simulink model "RefModel_Control"  (R2020b)
settings: Solver=ode1  StartTime=0.0  StopTime=1  FixedStep=0.012  MaxStep=Ts  RelTol=1e-3
settings Model: Creator=sl  LastModifiedBy=a4327481
settings DataIOCC: SaveOutput=off  SaveTime=off
settings OptimizationCC: DefaultParameterBehavior=Inlined  EnhancedBackFolding=on  PassReuseOutputArgsAs=Individual arguments  ZeroExternalMemoryAtStartup=off  ZeroInternalMemoryAtStartup=off  OptimizeBlockOrder=speed  DifferentSizesBufferReuse=on  OptimizationCustomize=off  EfficientTunableParamExpr=on
settings DebuggingCC: InheritedTsInSrcMsg=none  ParameterPrecisionLossMsg=none  ParameterTunabilityLossMsg=error  UnconnectedInputMsg=none  UnconnectedOutputMsg=none  UnconnectedLineMsg=none
settings HardwareCC: ProdBitPerPointer=32  ProdBitPerSizeT=32  ProdBitPerPtrDiffT=32  ProdLargestAtomicInteger=Long  ProdLargestAtomicFloat=Double  ProdWordSize=32  ProdHWDeviceType=ARM Compatible->ARM Cortex
settings ModelReferenceCC: ParallelModelReferenceMATLABWorkerInit=Copy Base Workspace  ModelReferenceNumInstancesAllowed=Single
settings SFSimCC: MATLABDynamicMemAlloc=off
settings RTWCC: Description=Embedded Coder  SystemTargetFile=ert.tlc  GenCodeOnly=on  PackageGeneratedCodeAndArtifacts=on  TemplateMakefile=ert_default_tmf  GenerateReport=on  IncludeHyperlinkInReport=on  LaunchReport=on  GenerateTraceInfo=on  GenerateTraceReport=on  GenerateTraceReportSl=on  GenerateTraceReportSf=on  GenerateTraceReportEml=on
settings CodeAppCC: ForceParamTrailComments=on  IgnoreCustomStorageClasses=off  MaxIdLength=48  OperatorAnnotations=on  SimulinkDataObjDesc=on  SFDataObjDesc=on  MATLABFcnDesc=on  InsertBlockDesc=on  MATLABSourceComments=on
settings ERTTargetCC: TargetLangStandard=C99 (ISO)  GenerateSampleERTMain=on  LogVarNameModifier=none  SupportVariableSizeSignals=on  InlinedParameterPlacement=NonHierarchical  ERTCustomFileTemplate=example_file_process.tlc  ERTFilePackagingFormat=Compact

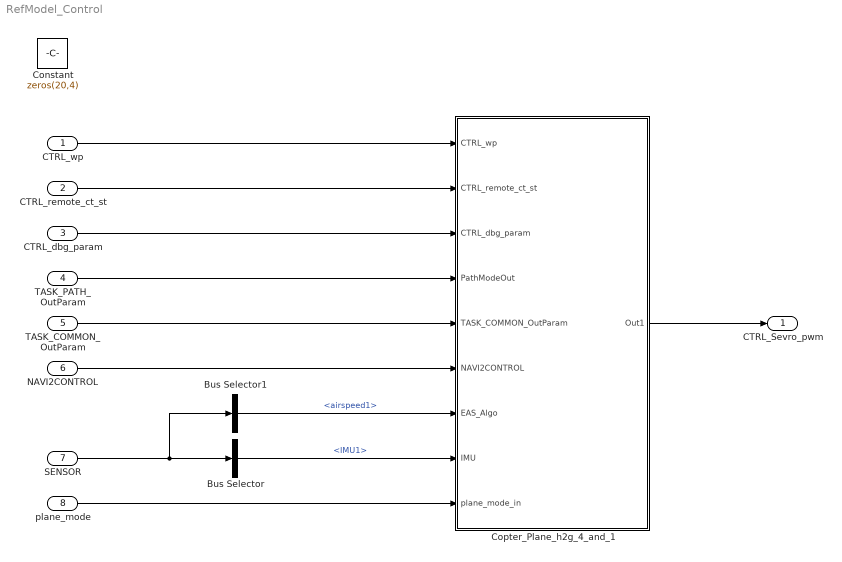
== system RefModel_Control ==
  CTRL_wp : Inport  BusOutputAsStruct=on
  CTRL_remote_ct_st : Inport  Port=2  OutDataTypeStr=Bus: BUS_CTRL_remote_ct_st  BusOutputAsStruct=on
  CTRL_dbg_param : Inport  Port=3  OutDataTypeStr=Bus: BUS_CTRL_dbg_param  BusOutputAsStruct=on
  TASK_PATH_OutParam : Inport  Port=4  OutDataTypeStr=Bus: BUS_TASK_PATH_OutParam  BusOutputAsStruct=on
  TASK_COMMON_OutParam : Inport  Port=5  OutDataTypeStr=Bus: BUS_TASK_COMMON_OutParam  BusOutputAsStruct=on
  NAVI2CONTROL : Inport  Port=6  OutDataTypeStr=Bus: BUS_TO_CONTROL  BusOutputAsStruct=on
  SENSOR : Inport  Port=7  OutDataTypeStr=Bus: BUS_SENSOR
  plane_mode : Inport  Port=8  OutDataTypeStr=Enum: ENUM_plane_mode
  Bus Selector : BusSelector  OutputSignals=IMU1
  Bus Selector1 : BusSelector  OutputSignals=airspeed1
  Constant : Constant  Value=zeros(20,4)
  Copter_Plane_h2g_4_and_1 : Subsystem
  CTRL_Sevro_pwm : Outport  OutDataTypeStr=Bus: BUS_CTRL_SRV_Channel
  wires:
  NAVI2CONTROL/1 -> Copter_Plane_h2g_4_and_1/6(NAVI2CONTROL)
  Copter_Plane_h2g_4_and_1/1(Out1) -> CTRL_Sevro_pwm/1
  Bus Selector1/1 -> Copter_Plane_h2g_4_and_1/7(EAS_Algo)  "<airspeed1>"
  CTRL_dbg_param/1 -> Copter_Plane_h2g_4_and_1/3(CTRL_dbg_param)
  CTRL_remote_ct_st/1 -> Copter_Plane_h2g_4_and_1/2(CTRL_remote_ct_st)
  SENSOR/1 -> Bus Selector1/1, Bus Selector/1
  TASK_COMMON_OutParam/1 -> Copter_Plane_h2g_4_and_1/5(TASK_COMMON_OutParam)
  CTRL_wp/1 -> Copter_Plane_h2g_4_and_1/1(CTRL_wp)
  Bus Selector/1 -> Copter_Plane_h2g_4_and_1/8(IMU)  "<IMU1>"
  plane_mode/1 -> Copter_Plane_h2g_4_and_1/9(plane_mode_in)
  TASK_PATH_OutParam/1 -> Copter_Plane_h2g_4_and_1/4(PathModeOut)

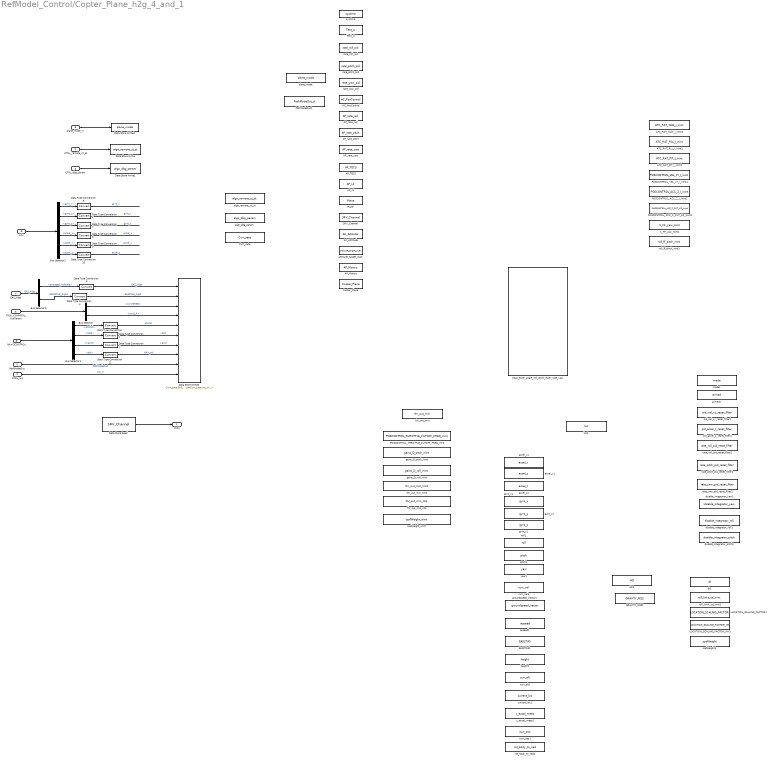
== system RefModel_Control/Copter_Plane_h2g_4_and_1 ==
  CTRL_wp : Inport
  CTRL_remote_ct_st : Inport  Port=2  OutDataTypeStr=Bus: BUS_CTRL_remote_ct_st
  CTRL_dbg_param : Inport  Port=3  OutDataTypeStr=Bus: BUS_CTRL_dbg_param
  PathModeOut : Inport  Port=4  OutDataTypeStr=Bus: BUS_TASK_PATH_OutParam
  TASK_COMMON_OutParam : Inport  Port=5  OutDataTypeStr=Bus: BUS_TASK_COMMON_OutParam
  NAVI2CONTROL : Inport  Port=6  OutDataTypeStr=Bus: BUS_TO_CONTROL
  EAS_Algo : Inport  Port=7  OutDataTypeStr=Bus: BUS_AIRSPEED
  IMU : Inport  Port=8  OutDataTypeStr=Bus: BUS_IMU
  plane_mode_in : Inport  Port=9
  AC_Attitude : DataStoreMemory  DataStoreName=AC_Attitude  ReadBeforeWriteMsg=warning  WriteAfterWriteMsg=warning  WriteAfterReadMsg=warning  InitialValue=AC_Attitude  ShowAdditionalParam=off  OutDataTypeStr=Bus: BUS_CTRL_AC_Attitude
  AC_PosControl : DataStoreMemory  DataStoreName=AC_PosControl  ReadBeforeWriteMsg=warning  WriteAfterWriteMsg=warning  WriteAfterReadMsg=warning  InitialValue=AC_PosControl  ShowAdditionalParam=off  OutDataTypeStr=Bus: BUS_CTRL_AC_PosControl
  AP_L1 : DataStoreMemory  DataStoreName=AP_L1  ReadBeforeWriteMsg=warning  WriteAfterWriteMsg=warning  WriteAfterReadMsg=warning  InitialValue=AP_L1  ShowAdditionalParam=off  OutDataTypeStr=Bus: BUS_CTRL_AP_L1
  AP_Motors : DataStoreMemory  DataStoreName=AP_Motors  ReadBeforeWriteMsg=warning  WriteAfterWriteMsg=warning  WriteAfterReadMsg=warning  InitialValue=AP_Motors  VectorParams1D=off  ShowAdditionalParam=off  OutDataTypeStr=Bus: BUS_CTRL_AP_Motors
  AP_TECS : DataStoreMemory  DataStoreName=AP_TECS  ReadBeforeWriteMsg=warning  WriteAfterWriteMsg=warning  WriteAfterReadMsg=warning  InitialValue=AP_TECS  ShowAdditionalParam=off  OutDataTypeStr=Bus: BUS_CTRL_AP_TECS
  AP_rate_pitch : DataStoreMemory  DataStoreName=AP_rate_pitch  ReadBeforeWriteMsg=warning  WriteAfterWriteMsg=warning  WriteAfterReadMsg=warning  InitialValue=AP_rate_pitch  ShowAdditionalParam=off  OutDataTypeStr=Bus: BUS_CTRL_AP_PID_pitch
  AP_rate_roll : DataStoreMemory  DataStoreName=AP_rate_roll  ReadBeforeWriteMsg=warning  WriteAfterWriteMsg=warning  WriteAfterReadMsg=warning  InitialValue=AP_rate_roll  ShowAdditionalParam=off  OutDataTypeStr=Bus: BUS_CTRL_AP_PID_roll
  AP_rate_yaw : DataStoreMemory  DataStoreName=AP_rate_yaw  ReadBeforeWriteMsg=warning  WriteAfterWriteMsg=warning  WriteAfterReadMsg=warning  InitialValue=AP_rate_yaw  ShowAdditionalParam=off  OutDataTypeStr=Bus: BUS_CTRL_AP_PID_yaw
  ATC_RAT_PIT_I_inint1 : DataStoreMemory  DataStoreName=ATC_RAT_PIT_I_inint  ReadBeforeWriteMsg=warning  WriteAfterWriteMsg=warning  WriteAfterReadMsg=warning  InitialValue=ATC_RAT_PIT_I_inint  VectorParams1D=off  ShowAdditionalParam=off  OutDataTypeStr=double
  ATC_RAT_RLL_I_inint1 : DataStoreMemory  DataStoreName=ATC_RAT_RLL_I_inint  ReadBeforeWriteMsg=warning  WriteAfterWriteMsg=warning  WriteAfterReadMsg=warning  InitialValue=ATC_RAT_RLL_I_inint  VectorParams1D=off  ShowAdditionalParam=off  OutDataTypeStr=double
  ATC_RAT_YAW_I_inint1 : DataStoreMemory  DataStoreName=ATC_RAT_YAW_I_inint  ReadBeforeWriteMsg=warning  WriteAfterWriteMsg=warning  WriteAfterReadMsg=warning  InitialValue=ATC_RAT_YAW_I_inint  VectorParams1D=off  ShowAdditionalParam=off  OutDataTypeStr=double
  Bus Selector : BusSelector  OutputSignals=curVelNED,curLLA
  Bus Selector1 : BusSelector  OutputSignals=pitchd,rolld,yawd,alt
  Bus Selector2 : BusSelector  OutputSignals=gyro_x,gyro_y,gyro_z,accel_x,accel_y,accel_z
  Bus Selector3 : BusSelector  OutputSignals=airspeed_indicate,EAS2TAS_Algo
  Copter_Plane : DataStoreMemory  DataStoreName=Copter_Plane  ReadBeforeWriteMsg=warning  WriteAfterWriteMsg=warning  WriteAfterReadMsg=warning  InitialValue=Copter_Plane  VectorParams1D=off  ShowAdditionalParam=off  OutDataTypeStr=Bus: BUS_CTRL_Copter_Plane
  Curr_sate : DataStoreMemory  DataStoreName=Curr_sate  ReadBeforeWriteMsg=warning  WriteAfterWriteMsg=warning  WriteAfterReadMsg=warning  InitialValue=Curr_sate  VectorParams1D=off  ShowAdditionalParam=off  OutDataTypeStr=Bus: BUS_CTRL_Curr_sate
  Data Store Read : DataStoreRead  DataStoreName=SRV_Channel
  Data Store Write : DataStoreWrite  DataStoreName=algo_remote_ct_st
  Data Store Write1 : DataStoreWrite  DataStoreName=algo_dbg_param
  Data Store Write2 : DataStoreWrite  DataStoreName=Curr_sate  DataStoreElements=Curr_sate.EAS_Algo#Curr_sate.EAS2TAS_Algo#Curr_sate.curVelNED(:,:)#Curr_sate.curLLA(:,:)#Curr_sate.pitchd#Curr_sate.rolld#Curr_sate.yawd#Curr_sate.NAV_alt#Curr_sate.PathModeOut#Curr_sate.wp_in(:,:)
  Data Store Write3 : DataStoreWrite  DataStoreName=plane_mode
  Data Type Conversion{,1..11} (12 alike) : DataTypeConversion
  EAS2TAS1 : DataStoreMemory  DataStoreName=EAS2TAS  ReadBeforeWriteMsg=warning  WriteAfterWriteMsg=warning  WriteAfterReadMsg=warning  InitialValue=EAS2TAS  VectorParams1D=off  ShowAdditionalParam=off  OutDataTypeStr=double
  GRAVITY_MSS1 : DataStoreMemory  DataStoreName=GRAVITY_MSS  ReadBeforeWriteMsg=warning  WriteAfterWriteMsg=warning  WriteAfterReadMsg=warning  InitialValue=GRAVITY_MSS  VectorParams1D=off  ShowAdditionalParam=off  OutDataTypeStr=double
  HD1 : DataStoreMemory  DataStoreName=HD  ReadBeforeWriteMsg=warning  WriteAfterWriteMsg=warning  WriteAfterReadMsg=warning  InitialValue=HD  ShowAdditionalParam=off  OutDataTypeStr=double
  K_FF_yaw_inint1 : DataStoreMemory  DataStoreName=K_FF_yaw_inint  ReadBeforeWriteMsg=warning  WriteAfterWriteMsg=warning  WriteAfterReadMsg=warning  InitialValue=K_FF_yaw_inint  VectorParams1D=off  ShowAdditionalParam=off  OutDataTypeStr=double
  LOCATION_SCALING_FACTOR1 : DataStoreMemory  DataStoreName=LOCATION_SCALING_FACTOR  ReadBeforeWriteMsg=warning  WriteAfterWriteMsg=warning  WriteAfterReadMsg=warning  InitialValue=LOCATION_SCALING_FACTOR  VectorParams1D=off  ShowAdditionalParam=off  OutDataTypeStr=double
  LOCATION_SCALING_FACTOR_INV1 : DataStoreMemory  DataStoreName=LOCATION_SCALING_FACTOR_INV  ReadBeforeWriteMsg=warning  WriteAfterWriteMsg=warning  WriteAfterReadMsg=warning  InitialValue=LOCATION_SCALING_FACTOR_INV  VectorParams1D=off  ShowAdditionalParam=off  OutDataTypeStr=double
  POSCONTROL_ACC_Z_FILT_HZ_inint1 : DataStoreMemory  DataStoreName=POSCONTROL_ACC_Z_FILT_HZ_inint  ReadBeforeWriteMsg=warning  WriteAfterWriteMsg=warning  WriteAfterReadMsg=warning  InitialValue=POSCONTROL_ACC_Z_FILT_HZ_inint  VectorParams1D=off  ShowAdditionalParam=off  OutDataTypeStr=double
  POSCONTROL_ACC_Z_I_inint1 : DataStoreMemory  DataStoreName=POSCONTROL_ACC_Z_I_inint  ReadBeforeWriteMsg=warning  WriteAfterWriteMsg=warning  WriteAfterReadMsg=warning  InitialValue=POSCONTROL_ACC_Z_I_inint  VectorParams1D=off  ShowAdditionalParam=off  OutDataTypeStr=double
  POSCONTROL_THROTTLE_CUTOFF_FREQ_inint : DataStoreMemory  DataStoreName=POSCONTROL_THROTTLE_CUTOFF_FREQ_inint  ReadBeforeWriteMsg=warning  WriteAfterWriteMsg=warning  WriteAfterReadMsg=warning  InitialValue=POSCONTROL_THROTTLE_CUTOFF_FREQ_inint  VectorParams1D=off  ShowAdditionalParam=off  OutDataTypeStr=double
  POSCONTROL_VEL_XY_I_inint1 : DataStoreMemory  DataStoreName=POSCONTROL_VEL_XY_I_inint  ReadBeforeWriteMsg=warning  WriteAfterWriteMsg=warning  WriteAfterReadMsg=warning  InitialValue=POSCONTROL_VEL_XY_I_inint  VectorParams1D=off  ShowAdditionalParam=off  OutDataTypeStr=double
  PathModeOut1 : DataStoreMemory  DataStoreName=PathModeOut_sl  ReadBeforeWriteMsg=warning  WriteAfterWriteMsg=warning  WriteAfterReadMsg=warning  InitialValue=PathModeOut_sl  VectorParams1D=off  ShowAdditionalParam=off  OutDataTypeStr=Bus: BUS_TASK_PATH_OutParam
  Plane : DataStoreMemory  DataStoreName=Plane  ReadBeforeWriteMsg=warning  WriteAfterWriteMsg=warning  WriteAfterReadMsg=warning  InitialValue=Plane  ShowAdditionalParam=off  OutDataTypeStr=Bus: BUS_CTRL_Plane
  SRV_Channel : DataStoreMemory  DataStoreName=SRV_Channel  ReadBeforeWriteMsg=warning  WriteAfterWriteMsg=warning  WriteAfterReadMsg=warning  InitialValue=SRV_Channel  ShowAdditionalParam=off  OutDataTypeStr=Bus: BUS_CTRL_SRV_Channel
  Test_w : DataStoreMemory  DataStoreName=Test_w  ReadBeforeWriteMsg=warning  WriteAfterWriteMsg=warning  WriteAfterReadMsg=warning  InitialValue=Test_w  ShowAdditionalParam=off  OutDataTypeStr=Bus: BUS_CTRL_Test_w
  accel_x1 : DataStoreMemory  DataStoreName=accel_x  ReadBeforeWriteMsg=warning  WriteAfterWriteMsg=warning  WriteAfterReadMsg=warning  InitialValue=accel_x  ShowAdditionalParam=off  OutDataTypeStr=double
  accel_y1 : DataStoreMemory  DataStoreName=accel_y  ReadBeforeWriteMsg=warning  WriteAfterWriteMsg=warning  WriteAfterReadMsg=warning  InitialValue=accel_y  ShowAdditionalParam=off  OutDataTypeStr=double
  accel_z1 : DataStoreMemory  DataStoreName=accel_z  ReadBeforeWriteMsg=warning  WriteAfterWriteMsg=warning  WriteAfterReadMsg=warning  InitialValue=accel_z  ShowAdditionalParam=off  OutDataTypeStr=double
  algo_dbg_param : DataStoreMemory  DataStoreName=algo_dbg_param  ReadBeforeWriteMsg=warning  WriteAfterWriteMsg=warning  WriteAfterReadMsg=warning  InitialValue=algo_dbg_param  VectorParams1D=off  ShowAdditionalParam=off  OutDataTypeStr=Bus: BUS_CTRL_dbg_param
  algo_remote_ct_st : DataStoreMemory  DataStoreName=algo_remote_ct_st  ReadBeforeWriteMsg=warning  WriteAfterWriteMsg=warning  WriteAfterReadMsg=warning  InitialValue=algo_remote_ct_st  VectorParams1D=off  ShowAdditionalParam=off  OutDataTypeStr=Bus:BUS_CTRL_remote_ct_st
  armed1 : DataStoreMemory  DataStoreName=armed  ReadBeforeWriteMsg=warning  WriteAfterWriteMsg=warning  WriteAfterReadMsg=warning  InitialValue=armed  VectorParams1D=off  ShowAdditionalParam=off  OutDataTypeStr=double
  aspeed1 : DataStoreMemory  DataStoreName=aspeed  ReadBeforeWriteMsg=warning  WriteAfterWriteMsg=warning  WriteAfterReadMsg=warning  InitialValue=aspeed  ShowAdditionalParam=off  OutDataTypeStr=double
  attitude_target_quat : DataStoreMemory  DataStoreName=attitude_target_quat  ReadBeforeWriteMsg=warning  WriteAfterWriteMsg=warning  WriteAfterReadMsg=warning  InitialValue=attitude_target_quat  VectorParams1D=off  ShowAdditionalParam=off  OutDataTypeStr=double
  curr_alt1 : DataStoreMemory  DataStoreName=curr_alt  ReadBeforeWriteMsg=warning  WriteAfterWriteMsg=warning  WriteAfterReadMsg=warning  InitialValue=curr_alt  VectorParams1D=off  ShowAdditionalParam=off  OutDataTypeStr=double
  curr_pos1 : DataStoreMemory  DataStoreName=curr_pos  ReadBeforeWriteMsg=warning  WriteAfterWriteMsg=warning  WriteAfterReadMsg=warning  InitialValue=curr_pos  ShowAdditionalParam=off  OutDataTypeStr=double
  curr_vel1 : DataStoreMemory  DataStoreName=curr_vel  ReadBeforeWriteMsg=warning  WriteAfterWriteMsg=warning  WriteAfterReadMsg=warning  InitialValue=curr_vel  VectorParams1D=off  ShowAdditionalParam=off  OutDataTypeStr=double
  current_loc1 : DataStoreMemory  DataStoreName=current_loc  ReadBeforeWriteMsg=warning  WriteAfterWriteMsg=warning  WriteAfterReadMsg=warning  InitialValue=current_loc  VectorParams1D=off  ShowAdditionalParam=off  OutDataTypeStr=double
  disable_integrator_pitch1 : DataStoreMemory  DataStoreName=disable_integrator_pitch  ReadBeforeWriteMsg=warning  WriteAfterWriteMsg=warning  WriteAfterReadMsg=warning  InitialValue=disable_integrator_pitch  ShowAdditionalParam=off  OutDataTypeStr=double
  disable_integrator_roll1 : DataStoreMemory  DataStoreName=disable_integrator_roll  ReadBeforeWriteMsg=warning  WriteAfterWriteMsg=warning  WriteAfterReadMsg=warning  InitialValue=disable_integrator_roll  ShowAdditionalParam=off  OutDataTypeStr=double
  disable_integrator_yaw1 : DataStoreMemory  DataStoreName=disable_integrator_yaw  ReadBeforeWriteMsg=warning  WriteAfterWriteMsg=warning  WriteAfterReadMsg=warning  InitialValue=disable_integrator_yaw  ShowAdditionalParam=off  OutDataTypeStr=double
  dt1 : DataStoreMemory  DataStoreName=dt  ReadBeforeWriteMsg=warning  WriteAfterWriteMsg=warning  WriteAfterReadMsg=warning  InitialValue=dt  ShowAdditionalParam=off  OutDataTypeStr=double
  gains_D_pitch_inint : DataStoreMemory  DataStoreName=gains_D_pitch_inint  ReadBeforeWriteMsg=warning  WriteAfterWriteMsg=warning  WriteAfterReadMsg=warning  InitialValue=gains_D_pitch_inint  VectorParams1D=off  ShowAdditionalParam=off  OutDataTypeStr=double
  gains_D_roll_inint : DataStoreMemory  DataStoreName=gains_D_roll_inint  ReadBeforeWriteMsg=warning  WriteAfterWriteMsg=warning  WriteAfterReadMsg=warning  InitialValue=gains_D_roll_inint  VectorParams1D=off  ShowAdditionalParam=off  OutDataTypeStr=double
  groundspeed_vector1 : DataStoreMemory  DataStoreName=groundspeed_vector  ReadBeforeWriteMsg=warning  WriteAfterWriteMsg=warning  WriteAfterReadMsg=warning  InitialValue=groundspeed_vector  VectorParams1D=off  ShowAdditionalParam=off  OutDataTypeStr=double
  gyro_x1 : DataStoreMemory  DataStoreName=gyro_x  ReadBeforeWriteMsg=warning  WriteAfterWriteMsg=warning  WriteAfterReadMsg=warning  InitialValue=gyro_x  ShowAdditionalParam=off  OutDataTypeStr=double
  gyro_y1 : DataStoreMemory  DataStoreName=gyro_y  ReadBeforeWriteMsg=warning  WriteAfterWriteMsg=warning  WriteAfterReadMsg=warning  InitialValue=gyro_y  ShowAdditionalParam=off  OutDataTypeStr=double
  gyro_z1 : DataStoreMemory  DataStoreName=gyro_z  ReadBeforeWriteMsg=warning  WriteAfterWriteMsg=warning  WriteAfterReadMsg=warning  InitialValue=gyro_z  ShowAdditionalParam=off  OutDataTypeStr=double
  height1 : DataStoreMemory  DataStoreName=height  ReadBeforeWriteMsg=warning  WriteAfterWriteMsg=warning  WriteAfterReadMsg=warning  InitialValue=height  VectorParams1D=off  ShowAdditionalParam=off  OutDataTypeStr=double
  input_euler_angle_roll_pitch_euler_rate_yaw : MATLAB Function  TreatAsAtomicUnit=on
  loc1 : DataStoreMemory  DataStoreName=loc  ReadBeforeWriteMsg=warning  WriteAfterWriteMsg=warning  WriteAfterReadMsg=warning  InitialValue=loc  VectorParams1D=off  ShowAdditionalParam=off  OutDataTypeStr=Bus: BUS_CTRL_wp
  mode1 : DataStoreMemory  DataStoreName=mode  ReadBeforeWriteMsg=warning  WriteAfterWriteMsg=warning  WriteAfterReadMsg=warning  InitialValue=mode  VectorParams1D=off  ShowAdditionalParam=off  OutDataTypeStr=double
  pid_accel_z_reset_filter1 : DataStoreMemory  DataStoreName=pid_accel_z_reset_filter  ReadBeforeWriteMsg=warning  WriteAfterWriteMsg=warning  WriteAfterReadMsg=warning  InitialValue=pid_accel_z_reset_filter  VectorParams1D=off  ShowAdditionalParam=off  OutDataTypeStr=double
  pid_vel_xy_reset_filter1 : DataStoreMemory  DataStoreName=pid_vel_xy_reset_filter  ReadBeforeWriteMsg=warning  WriteAfterWriteMsg=warning  WriteAfterReadMsg=warning  InitialValue=pid_vel_xy_reset_filter  VectorParams1D=off  ShowAdditionalParam=off  OutDataTypeStr=double
  pitch1 : DataStoreMemory  DataStoreName=pitch  ReadBeforeWriteMsg=warning  WriteAfterWriteMsg=warning  WriteAfterReadMsg=warning  InitialValue=pitch  ShowAdditionalParam=off  OutDataTypeStr=double
  plane_mode : DataStoreMemory  DataStoreName=plane_mode  ReadBeforeWriteMsg=warning  WriteAfterWriteMsg=warning  WriteAfterReadMsg=warning  InitialValue=plane_mode  VectorParams1D=off  ShowAdditionalParam=off  OutDataTypeStr=Enum: ENUM_plane_mode
  rate_pitch_pid : DataStoreMemory  DataStoreName=rate_pitch_pid  ReadBeforeWriteMsg=warning  WriteAfterWriteMsg=warning  WriteAfterReadMsg=warning  InitialValue=rate_pitch_pid  ShowAdditionalParam=off  OutDataTypeStr=Bus: BUS_CTRL_PID
  rate_pitch_pid_reset_filter1 : DataStoreMemory  DataStoreName=rate_pitch_pid_reset_filter  ReadBeforeWriteMsg=warning  WriteAfterWriteMsg=warning  WriteAfterReadMsg=warning  InitialValue=rate_pitch_pid_reset_filter  VectorParams1D=off  ShowAdditionalParam=off  OutDataTypeStr=double
  rate_roll_pid : DataStoreMemory  DataStoreName=rate_roll_pid  ReadBeforeWriteMsg=warning  WriteAfterWriteMsg=warning  WriteAfterReadMsg=warning  InitialValue=rate_roll_pid  ShowAdditionalParam=off  OutDataTypeStr=Bus: BUS_CTRL_PID
  rate_roll_pid_reset_filter1 : DataStoreMemory  DataStoreName=rate_roll_pid_reset_filter  ReadBeforeWriteMsg=warning  WriteAfterWriteMsg=warning  WriteAfterReadMsg=warning  InitialValue=rate_roll_pid_reset_filter  VectorParams1D=off  ShowAdditionalParam=off  OutDataTypeStr=double
  rate_yaw_pid : DataStoreMemory  DataStoreName=rate_yaw_pid  ReadBeforeWriteMsg=warning  WriteAfterWriteMsg=warning  WriteAfterReadMsg=warning  InitialValue=rate_yaw_pid  ShowAdditionalParam=off  OutDataTypeStr=Bus: BUS_CTRL_PID
  rate_yaw_pid_reset_filter1 : DataStoreMemory  DataStoreName=rate_yaw_pid_reset_filter  ReadBeforeWriteMsg=warning  WriteAfterWriteMsg=warning  WriteAfterReadMsg=warning  InitialValue=rate_yaw_pid_reset_filter  VectorParams1D=off  ShowAdditionalParam=off  OutDataTypeStr=double
  roll1 : DataStoreMemory  DataStoreName=roll  ReadBeforeWriteMsg=warning  WriteAfterWriteMsg=warning  WriteAfterReadMsg=warning  InitialValue=roll  ShowAdditionalParam=off  OutDataTypeStr=double
  roll_ff_pitch_inint1 : DataStoreMemory  DataStoreName=roll_ff_pitch_inint  ReadBeforeWriteMsg=warning  WriteAfterWriteMsg=warning  WriteAfterReadMsg=warning  InitialValue=roll_ff_pitch_inint  VectorParams1D=off  ShowAdditionalParam=off  OutDataTypeStr=double
  roll_limit_cd_inint1 : DataStoreMemory  DataStoreName=roll_limit_cd_inint  ReadBeforeWriteMsg=warning  WriteAfterWriteMsg=warning  WriteAfterReadMsg=warning  InitialValue=roll_limit_cd_inint  ShowAdditionalParam=off  OutDataTypeStr=double
  rot_body_to_ned1 : DataStoreMemory  DataStoreName=rot_body_to_ned  ReadBeforeWriteMsg=warning  WriteAfterWriteMsg=warning  WriteAfterReadMsg=warning  InitialValue=rot_body_to_ned  VectorParams1D=off  ShowAdditionalParam=off  OutDataTypeStr=double
  spdWeight1 : DataStoreMemory  DataStoreName=spdWeight  ReadBeforeWriteMsg=warning  WriteAfterWriteMsg=warning  WriteAfterReadMsg=warning  InitialValue=spdWeight  VectorParams1D=off  ShowAdditionalParam=off  OutDataTypeStr=double
  spdWeight_inint : DataStoreMemory  DataStoreName=spdWeight_inint  ReadBeforeWriteMsg=warning  WriteAfterWriteMsg=warning  WriteAfterReadMsg=warning  InitialValue=spdWeight_inint  VectorParams1D=off  ShowAdditionalParam=off  OutDataTypeStr=double
  systime : DataStoreMemory  DataStoreName=systime  ReadBeforeWriteMsg=warning  WriteAfterWriteMsg=warning  WriteAfterReadMsg=warning  InitialValue=systime  ShowAdditionalParam=off  OutDataTypeStr=double
  thr_out_min : DataStoreMemory  DataStoreName=thr_out_min  ReadBeforeWriteMsg=warning  WriteAfterWriteMsg=warning  WriteAfterReadMsg=warning  InitialValue=thr_out_min  VectorParams1D=off  ShowAdditionalParam=off  OutDataTypeStr=double
  thr_out_min_c2p : DataStoreMemory  DataStoreName=thr_out_min_c2p  ReadBeforeWriteMsg=warning  WriteAfterWriteMsg=warning  WriteAfterReadMsg=warning  InitialValue=thr_out_min_c2p  VectorParams1D=off  ShowAdditionalParam=off  OutDataTypeStr=double
  thr_out_min_inint : DataStoreMemory  DataStoreName=thr_out_min_inint  ReadBeforeWriteMsg=warning  WriteAfterWriteMsg=warning  WriteAfterReadMsg=warning  InitialValue=thr_out_min_inint  VectorParams1D=off  ShowAdditionalParam=off  OutDataTypeStr=double
  yaw1 : DataStoreMemory  DataStoreName=yaw  ReadBeforeWriteMsg=warning  WriteAfterWriteMsg=warning  WriteAfterReadMsg=warning  InitialValue=yaw  VectorParams1D=off  ShowAdditionalParam=off  OutDataTypeStr=double
  z_accel_meas1 : DataStoreMemory  DataStoreName=z_accel_meas  ReadBeforeWriteMsg=warning  WriteAfterWriteMsg=warning  WriteAfterReadMsg=warning  InitialValue=z_accel_meas  VectorParams1D=off  ShowAdditionalParam=off  OutDataTypeStr=double
  Out1 : Outport  OutDataTypeStr=Bus: BUS_CTRL_SRV_Channel
  wires:
  Data Type Conversion9/1 -> ?  "accel_y"
  Data Type Conversion10/1 -> ?  "accel_z"
  Data Type Conversion5/1 -> ?  "gyro_x"
  Data Type Conversion11/1 -> Data Store Write2/8  "NAV_alt"
  Bus Selector1/4 -> Data Type Conversion11/1  "<alt>"
  Bus Selector3/1 -> Data Type Conversion3/1  "<airspeed_indicate>"
  CTRL_dbg_param/1 -> Data Store Write1/1
  Data Type Conversion6/1 -> ?  "gyro_y"
  Data Type Conversion3/1 -> Data Store Write2/1  "EAS_Algo"
  Data Type Conversion4/1 -> Data Store Write2/2  "EAS2TAS_Algo"
  Bus Selector1/3 -> Data Type Conversion2/1  "<yawd>"
  CTRL_wp/1 -> Data Store Write2/10  "wp_in"
  Bus Selector2/1 -> Data Type Conversion5/1  "<gyro_x>"
  Bus Selector3/2 -> Data Type Conversion4/1  "<EAS2TAS_Algo>"
  Data Type Conversion/1 -> Data Store Write2/5  "pitchd"
  Data Type Conversion1/1 -> Data Store Write2/6  "rolld"
  Bus Selector1/1 -> Data Type Conversion/1  "<pitchd>"
  Data Type Conversion2/1 -> Data Store Write2/7  "yawd"
  Bus Selector/1 -> Data Store Write2/3  "<curVelNED>"
  Bus Selector1/2 -> Data Type Conversion1/1  "<rolld>"
  Bus Selector2/5 -> Data Type Conversion9/1  "<accel_y>"
  plane_mode_in/1 -> Data Store Write3/1
  CTRL_remote_ct_st/1 -> Data Store Write/1
  Bus Selector2/3 -> Data Type Conversion7/1  "<gyro_z>"
  Data Type Conversion8/1 -> ?  "accel_x"
  EAS_Algo/1 -> Bus Selector3/1  "EAS_Algo"
  NAVI2CONTROL/1 -> Bus Selector1/1
  Bus Selector/2 -> Data Store Write2/4  "<curLLA>"
  IMU/1 -> Bus Selector2/1
  Data Type Conversion7/1 -> ?  "gyro_z"
  Bus Selector2/4 -> Data Type Conversion8/1  "<accel_x>"
  TASK_COMMON_OutParam/1 -> Bus Selector/1
  PathModeOut/1 -> Data Store Write2/9  "PathModeOut"
  Bus Selector2/6 -> Data Type Conversion10/1  "<accel_z>"
  Bus Selector2/2 -> Data Type Conversion6/1  "<gyro_y>"
  Data Store Read/1 -> Out1/1

== matlab function RefModel_Control/Copter_Plane_h2g_4_and_1/input_euler_angle_roll_pitch_euler_rate_yaw ==
  data: roll data_store_memory; pitch data_store_memory; aspeed data_store_memory; GRAVITY_MSS data_store_memory; HD data_store_memory; accel_y data_store_memory; rot_body_to_ned data_store_memory; EAS2TAS data_store_memory; height data_store_memory; spdWeight data_store_memory; groundspeed_vector data_store_memory; yaw data_store_memory; dt data_store_memory; roll_limit_cd_inint data_store_memory; accel_x data_store_memory; accel_z data_store_memory; LOCATION_SCALING_FACTOR_INV data_store_memory; curr_alt data_store_memory; curr_vel data_store_memory; z_accel_meas data_store_memory; pid_accel_z_reset_filter data_store_memory; curr_pos data_store_memory; pid_vel_xy_reset_filter data_store_memory; gyro_z data_store_memory; gyro_x data_store_memory; gyro_y data_store_memory; armed data_store_memory; mode data_store_memory; loc data_store_memory; disable_integrator_pitch data_store_memory; disable_integrator_roll data_store_memory; disable_integrator_yaw data_store_memory; PathModeOut_sl data_store_memory; roll_ff_pitch_inint data_store_memory; K_FF_yaw_inint data_store_memory; ATC_RAT_PIT_I_inint data_store_memory; ATC_RAT_RLL_I_inint data_store_memory; ATC_RAT_YAW_I_inint data_store_memory; thr_out_min data_store_memory; plane_mode data_store_memory; algo_remote_ct_st data_store_memory; algo_dbg_param data_store_memory; Curr_sate data_store_memory; gains_D_pitch_inint data_store_memory; gains_D_roll_inint data_store_memory; thr_out_min_inint data_store_memory; spdWeight_inint data_store_memory; thr_out_min_c2p data_store_memory; systime data_store_memory; Test_w data_store_memory; rate_pitch_pid data_store_memory; rate_roll_pid data_store_memory; rate_yaw_pid data_store_memory; AC_PosControl data_store_memory; AP_rate_roll data_store_memory; AP_rate_pitch data_store_memory; AP_rate_yaw data_store_memory; POSCONTROL_ACC_Z_I_inint data_store_memory; POSCONTROL_VEL_XY_I_inint data_store_memory; POSCONTROL_ACC_Z_FILT_HZ_inint data_store_memory; POSCONTROL_THROTTLE_CUTOFF_FREQ_inint data_store_memory; rate_pitch_pid_reset_filter data_store_memory; rate_roll_pid_reset_filter data_store_memory; rate_yaw_pid_reset_filter data_store_memory; AP_TECS data_store_memory; AP_L1 data_store_memory; Plane data_store_memory; SRV_Channel data_store_memory; AC_Attitude data_store_memory; attitude_target_quat data_store_memory; AP_Motors data_store_memory; Copter_Plane data_store_memory; LOCATION_SCALING_FACTOR data_store_memory; current_loc data_store_memory
function copter_plane_run
global plane_mode

run_remote();
load_Curr_sate();
loc_run();
% load_inint();
sin_step_test();
    switch plane_mode
        case ENUM_plane_mode.V1000
            run_V1000();
        case ENUM_plane_mode.V10
            run_V10();
        case ENUM_plane_mode.V10s
            run_V10s();
        case ENUM_plane_mode.V10_1
            run_V10();
        otherwise
            run_V10();
    end 
run_servo_pwm_adj();

end
